simulink model "linear_simulation_stabilization"  (R2023a)
settings: Solver=VariableStepAuto  StartTime=0.0  StopTime=1  RelTol=1e-3
undefined symbols (not defined in the file): A_front, A_side, b_front, b_side, C_out, init_cond, Ts
settings Model: Creator=ninj2  LastModifiedBy=morit
settings OptimizationCC: ReuseModelBlockBuffer=off

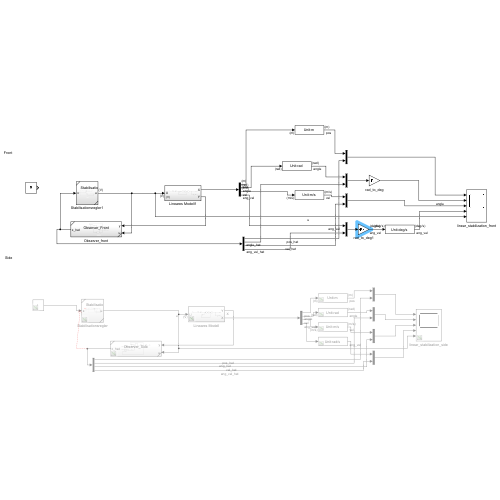
[thumbnail: Simulink's stored preview of the top-level diagram]
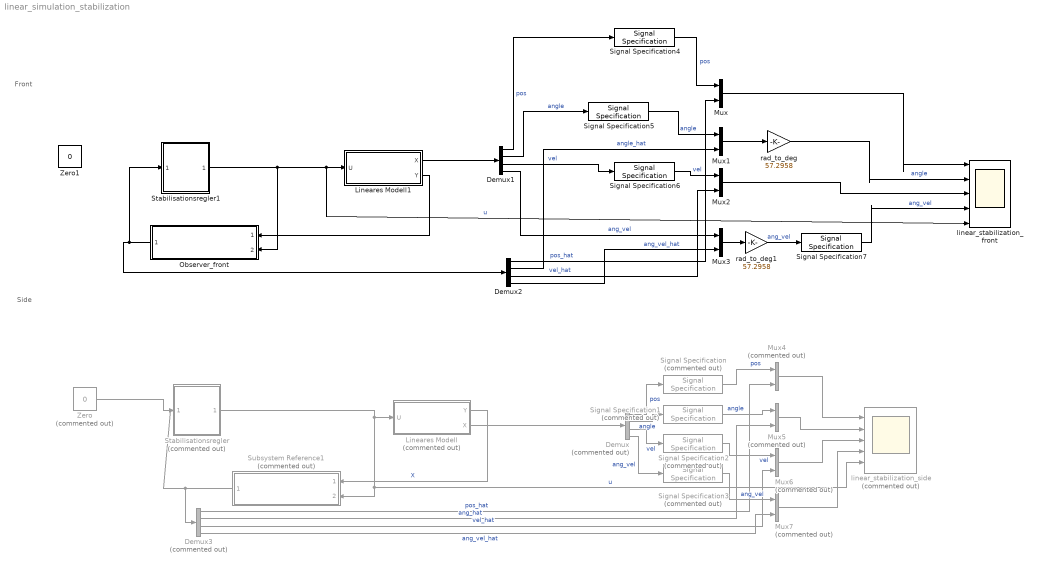
== system linear_simulation_stabilization ==
  note: Side
  note: Front
  Demux : Demux  Commented=on
  Demux1 : Demux
  Demux2 : Demux
  Demux3 : Demux  Commented=on
  Lineares Modell : Subsystem  Commented=on
  Lineares Modell1 : Subsystem
  Mux{,1..3} (4 alike) : Mux  Inputs=2
  Mux{4..7} (4 alike) : Mux  Commented=on  Inputs=2
  Observer_front : Subsystem  ReferencedSubsystem=Observer_Front
  Signal Specification : SignalSpecification  Commented=on  Unit=m
  Signal Specification1 : SignalSpecification  Commented=on  Unit=rad
  Signal Specification2 : SignalSpecification  Commented=on  Unit=m/s
  Signal Specification3 : SignalSpecification  Commented=on  Unit=rad/s
  Signal Specification4 : SignalSpecification  Unit=m
  Signal Specification5 : SignalSpecification  Unit=rad
  Signal Specification6 : SignalSpecification  Unit=m/s
  Signal Specification7 : SignalSpecification  Unit=deg/s
  Stabilisationsregler : Subsystem  Commented=on  ReferencedSubsystem=Stabilisationsregler_side
  Stabilisationsregler1 : Subsystem  ReferencedSubsystem=Stabilisationsregler_front
  Subsystem Reference1 : Subsystem  Commented=on  ReferencedSubsystem=Observer_Side
  Zero : Constant  Commented=on  Value=0  OutDataTypeStr=Inherit: Inherit via back propagation
  Zero1 : Constant  Value=0  OutDataTypeStr=Inherit: Inherit via back propagation
  linear_stabilization_front : Scope  NumInputPorts=5
  linear_stabilization_side : Scope  Commented=on  NumInputPorts=5
  rad_to_deg : Gain  Gain=57.2958
  rad_to_deg1 : Gain  Gain=57.2958
  wires:
  Lineares Modell/2(X) -> Demux/1
  Demux/1 -> Signal Specification/1  "pos"
  Demux/2 -> Signal Specification1/1  "angle"
  Demux/3 -> Signal Specification2/1  "vel"
  Demux/4 -> Signal Specification3/1  "ang_vel"
  Stabilisationsregler/1 -> linear_stabilization_side/5, Subsystem Reference1/2, Lineares Modell/1(U)  "u"
  Zero/1 -> Stabilisationsregler/1
  Lineares Modell1/1(X) -> Demux1/1
  Demux1/1 -> Signal Specification4/1  "pos"
  Demux1/3 -> Signal Specification6/1  "vel"
  Demux1/2 -> Signal Specification5/1  "angle"
  Demux1/4 -> Mux3/1  "ang_vel"
  Stabilisationsregler1/1 -> Observer_front/2, linear_stabilization_front/5, Lineares Modell1/1(U)  "u"
  Lineares Modell1/2(Y) -> Observer_front/1
  Signal Specification4/1 -> Mux/1  "pos"
  Demux2/1 -> Mux/2  "pos_hat"
  Mux/1 -> linear_stabilization_front/1
  Signal Specification5/1 -> Mux1/1  "angle"
  Demux2/2 -> Mux1/2  "angle_hat"
  Mux1/1 -> rad_to_deg/1
  Signal Specification6/1 -> Mux2/1  "vel"
  Demux2/3 -> Mux2/2  "vel_hat"
  Mux2/1 -> linear_stabilization_front/3
  Demux2/4 -> Mux3/2  "ang_vel_hat"
  Mux3/1 -> rad_to_deg1/1
  Observer_front/1 -> Stabilisationsregler1/1, Demux2/1
  Lineares Modell/1(Y) -> Subsystem Reference1/1  "X"
  Subsystem Reference1/1 -> Demux3/1
  Demux3/1 -> Mux4/2  "pos_hat"
  Demux3/2 -> Mux5/2  "ang_hat"
  Demux3/3 -> Mux6/2  "vel_hat"
  Demux3/4 -> Mux7/2  "ang_vel_hat"
  Signal Specification/1 -> Mux4/1  "pos"
  Signal Specification1/1 -> Mux5/1  "angle"
  Signal Specification2/1 -> Mux6/1  "vel"
  Signal Specification3/1 -> Mux7/1  "ang_vel"
  Mux4/1 -> linear_stabilization_side/1
  Mux5/1 -> linear_stabilization_side/2
  Mux6/1 -> linear_stabilization_side/3
  Mux7/1 -> linear_stabilization_side/4
  rad_to_deg/1 -> linear_stabilization_front/2  "angle"
  rad_to_deg1/1 -> Signal Specification7/1  "ang_vel"
  Signal Specification7/1 -> linear_stabilization_front/4  "ang_vel"

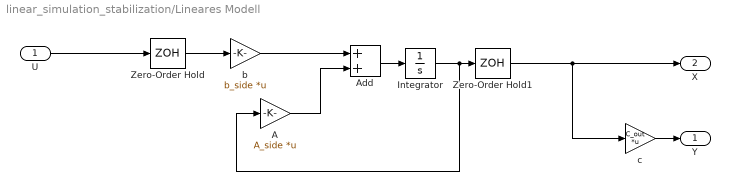
== system linear_simulation_stabilization/Lineares Modell ==
  U : Inport  Unit=V
  A : Gain  Gain=A_side  Multiplication=Matrix(K*u)
  Add : Sum
  Integrator : Integrator  InitialCondition=init_cond
  Zero-Order Hold : ZeroOrderHold  SampleTime=Ts
  Zero-Order Hold1 : ZeroOrderHold  SampleTime=Ts
  b : Gain  Gain=b_side  Multiplication=Matrix(K*u)
  c : Gain  Gain=C_out  Multiplication=Matrix(K*u)
  Y : Outport
  X : Outport  Port=2
  wires:
  A/1 -> Add/2
  Add/1 -> Integrator/1
  Integrator/1 -> A/1, Zero-Order Hold1/1
  c/1 -> Y/1
  Zero-Order Hold/1 -> b/1
  b/1 -> Add/1
  Zero-Order Hold1/1 -> c/1, X/1
  U/1 -> Zero-Order Hold/1

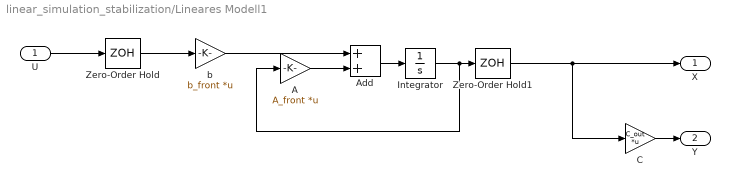
== system linear_simulation_stabilization/Lineares Modell1 ==
  U : Inport  Unit=V
  A : Gain  Gain=A_front  Multiplication=Matrix(K*u)
  Add : Sum
  C : Gain  Gain=C_out  Multiplication=Matrix(K*u)
  Integrator : Integrator  InitialCondition=init_cond
  Zero-Order Hold : ZeroOrderHold  SampleTime=Ts
  Zero-Order Hold1 : ZeroOrderHold  SampleTime=Ts
  b : Gain  Gain=b_front  Multiplication=Matrix(K*u)
  X : Outport
  Y : Outport  Port=2
  wires:
  A/1 -> Add/2
  Add/1 -> Integrator/1
  Integrator/1 -> A/1, Zero-Order Hold1/1
  C/1 -> Y/1
  Zero-Order Hold/1 -> b/1
  b/1 -> Add/1
  Zero-Order Hold1/1 -> C/1, X/1
  U/1 -> Zero-Order Hold/1
